simulink model "mpc_papermachine"  (R2021b)
settings: Solver=ode45  StartTime=0.0  StopTime=30.0  RelTol=1e-3  EnableMultiTasking=on
libraries: mpclib x1
settings Model: Creator=The MathWorks, Inc.  LastModifiedBy=Morteza-PC
settings SolverCC: AlgebraicLoopSolver=TrustRegion
settings DataIOCC: LimitDataPoints=on  SaveFormat=Array  ReturnWorkspaceOutputs=off  SignalLoggingName=sigsOut
settings OptimizationCC: ExpressionDepthLimit=2147483647  InitFltsAndDblsToZero=on  LifeSpan=inf
settings DebuggingCC: SaveWithParameterizedLinksMsg=none  UnderspecifiedInitializationDetection=Classic  MergeDetectMultiDrivingBlocksExec=none  CheckExecutionContextPreStartOutputMsg=on  SignalResolutionControl=TryResolveAllWithWarning  MultiTaskDSMMsg=warning  MultiTaskCondExecSysMsg=none  FcnCallInpInsideContextMsg=warning  StateNameClashWarn=warning  SFUnexpectedBacktrackingDiag=warning  SFNoUnconditionalDefaultTransitionDiag=warning  SFExecutionAtInitializationDiag=none  SFMachineParentedDataDiag=warning  ArithmeticOperatorsInVariantConditions=warning
settings HardwareCC: ProdBitPerPointer=32  ProdBitPerSizeT=32  ProdBitPerPtrDiffT=32  ProdLargestAtomicFloat=None  ProdIntDivRoundTo=Undefined  ProdEndianess=Unspecified  ProdWordSize=32  ProdHWDeviceType=32-bit Generic  TargetUnknown=on
settings ModelReferenceCC: PropagateSignalLabelsOutOfModel=off
settings SFSimCC: SimUseLocalCustomCode=off  CustomCodeUndefinedFunction=UseInterfaceOnly
settings RTWCC: RTWUseLocalCustomCode=off
settings CodeAppCC: StateflowObjectComments=on
settings GRTTargetCC: TargetFcnLib=ansi_tfl_tmw.mat  TargetLangStandard=C89/C90 (ANSI)  CombineOutputUpdateFcns=off  GRTInterface=on
settings ConfigComp: CovMetricSettings=dw  CovSaveCumulativeToWorkspaceVar=on  CovSaveSingleToWorkspaceVar=on  CovExternalEMLEnable=off  CovSFcnEnable=off

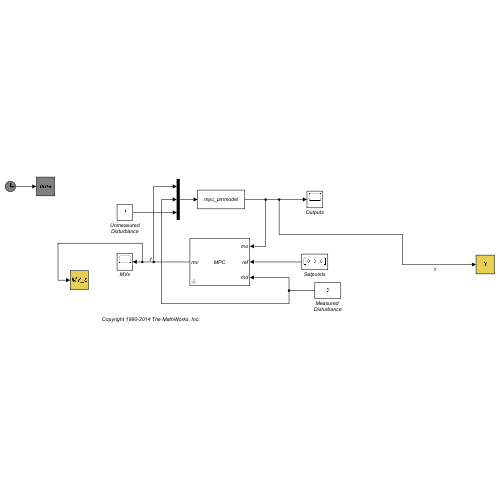
[thumbnail: Simulink's stored preview of the top-level diagram]
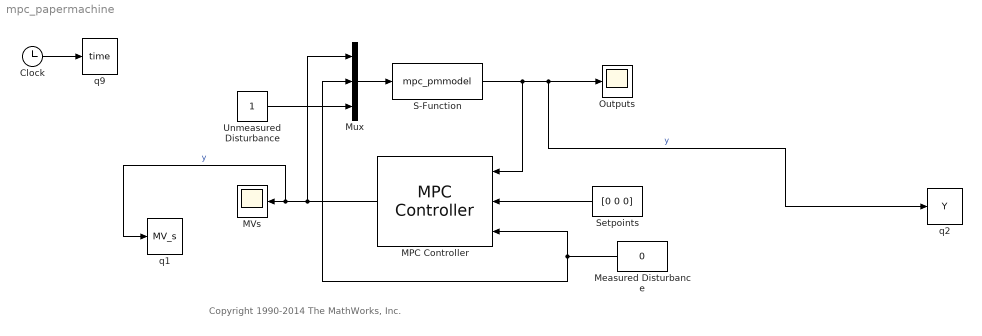
== system mpc_papermachine ==
  note: Copyright 1990-2014 The MathWorks, Inc.
  Clock : Clock
  MPC Controller : mpclib/MPC Controller  mpcobj=mpc1  x0=[]  is_multiple=0  enable_value=0  return_u0=off  updateMPCinCallerWorkspace=on  md_inport=on  mv_inport=off  uref_inport=off  return_cost=off  return_mvseq=off  return_qpstatus=off  return_xseq=off  return_state=off  return_ovseq=off  state_inport=off  umin_inport=off  umax_inport=off  ymin_inport=off  ymax_inport=off  cc_inport=off  ywt_inport=off  uwt_inport=off  duwt_inport=off  rhoeps_inport=off  pm_inport=off  MaximumP=10  HorizonChoice=FixedHorizon  n_ts=0.25  n_p=10  n_mv=2  n_md=1  n_ud=1  n_mo=3  n_uo=0  BlockDataType=double  SampleTimeInherited=off  switch_inport=off
  MVs : Scope
  Measured Disturbance : Constant  Value=0
  Mux : Mux  Inputs=3
  Outputs : Scope
  S-Function : S-Function  FunctionName=mpc_pmmodel  SFunctionDeploymentMode=off  EnableBusSupport=off
  Setpoints : Constant  Value=[0 0 0]
  Unmeasured Disturbance : Constant
  q1 : ToWorkspace  VariableName=MV_s  SampleTime=-1
      settings: Save2DSignal=2-D array (concatenate along first dimension)
  q2 : ToWorkspace  VariableName=Y  SampleTime=-1
  q9 : ToWorkspace  VariableName=time  SampleTime=-1
  wires:
  Setpoints/1 -> MPC Controller/2
  Measured Disturbance/1 -> Mux/2, MPC Controller/3
  Mux/1 -> S-Function/1
  Unmeasured Disturbance/1 -> Mux/3
  Clock/1 -> q9/1
  S-Function/1 -> q2/1, Outputs/1, MPC Controller/1  "y"
  MPC Controller/1 -> Mux/1, q1/1, MVs/1  "y"
